simulink model "case2"  (R2024b)
settings: Solver=FixedStepAuto  StartTime=0  StopTime=1  FixedStep=1e-7  RelTol=1e-3
values from neighbouring files (symbols this model uses):
  SG_D_1_D = 0.01056    [IEEE9_case_parameters.m]    (also in case1_parameters.m; case2_parameters.m; case3_parameters.m; case4_parameters.m)
  SG_D_1_EnableSaturation = 0    [IEEE9_case_parameters.m]    (also in case1_parameters.m; case2_parameters.m; case3_parameters.m; case4_parameters.m)
  SG_D_1_f0 = 60    [IEEE9_case_parameters.m]    (also in case1_parameters.m; case2_parameters.m; case3_parameters.m; case4_parameters.m)
  SG_D_1_H = 7.5    [IEEE9_case_parameters.m]    (also in case1_parameters.m; case2_parameters.m; case3_parameters.m; case4_parameters.m)
  SG_D_1_K_A = 20    [IEEE9_case_parameters.m]    (also in case1_parameters.m; case2_parameters.m; case3_parameters.m; case4_parameters.m)
  SG_D_1_K_E = 1.000000e+1    (= 10)    [IEEE9_case_parameters.m]    (also in case1_parameters.m; case2_parameters.m; case3_parameters.m; case4_parameters.m)
  SG_D_1_K_F = 2.363    [IEEE9_case_parameters.m]    (also in case1_parameters.m; case2_parameters.m; case3_parameters.m; case4_parameters.m)
  SG_D_1_K_s = 0.5    [IEEE9_case_parameters.m]    (also in case1_parameters.m = 5; case2_parameters.m = 5; case3_parameters.m = 5; case4_parameters.m = 5)
  SG_D_1_R_a = 0.001088    [IEEE9_case_parameters.m]    (also in case1_parameters.m; case2_parameters.m; case3_parameters.m; case4_parameters.m)
  SG_D_1_S_A = 1    [IEEE9_case_parameters.m]    (also in case1_parameters.m; case2_parameters.m; case3_parameters.m; case4_parameters.m)
  SG_D_1_S_B = 0.103    [IEEE9_case_parameters.m]    (also in case1_parameters.m; case2_parameters.m; case3_parameters.m; case4_parameters.m)
  SG_D_1_S_N = 10.659857    [IEEE9_case_parameters.m]    (also in case1_parameters.m; case2_parameters.m; case3_parameters.m; case4_parameters.m)
  SG_D_1_SpeedPara = 200    [IEEE9_case_parameters.m]    (also in case1_parameters.m; case2_parameters.m; case3_parameters.m; case4_parameters.m)
  SG_D_1_T_0 = 0.720173    [IEEE9_case_parameters.m]    (also in case1_parameters.m = 0.755522; case2_parameters.m = 0.808931; case3_parameters.m = 0.869402; case4_parameters.m = 0.729316)
  SG_D_1_T_1 = 0.3    [IEEE9_case_parameters.m]    (also in case1_parameters.m; case2_parameters.m; case3_parameters.m; case4_parameters.m)
  SG_D_1_T_2 = 0.05    [IEEE9_case_parameters.m]    (also in case1_parameters.m; case2_parameters.m; case3_parameters.m; case4_parameters.m)
  SG_D_1_T_3 = 0.02    [IEEE9_case_parameters.m]    (also in case1_parameters.m; case2_parameters.m; case3_parameters.m; case4_parameters.m)
  SG_D_1_T_4 = 0.005    [IEEE9_case_parameters.m]    (also in case1_parameters.m; case2_parameters.m; case3_parameters.m; case4_parameters.m)
  SG_D_1_T_A = 0.02    [IEEE9_case_parameters.m]    (also in case1_parameters.m; case2_parameters.m; case3_parameters.m; case4_parameters.m)
  SG_D_1_T_dd = 8.000000e+0    (= 8)    [IEEE9_case_parameters.m]    (also in case1_parameters.m; case2_parameters.m; case3_parameters.m; case4_parameters.m)
  SG_D_1_T_ddd = 0.04    [IEEE9_case_parameters.m]    (also in case1_parameters.m; case2_parameters.m; case3_parameters.m; case4_parameters.m)
  SG_D_1_T_E = 0.314    [IEEE9_case_parameters.m]    (also in case1_parameters.m; case2_parameters.m; case3_parameters.m; case4_parameters.m)
  SG_D_1_T_F = 0.35    [IEEE9_case_parameters.m]    (also in case1_parameters.m; case2_parameters.m; case3_parameters.m; case4_parameters.m)
  SG_D_1_T_qd = 0.8    [IEEE9_case_parameters.m]    (also in case1_parameters.m; case2_parameters.m; case3_parameters.m; case4_parameters.m)
  SG_D_1_T_qdd = 0.02    [IEEE9_case_parameters.m]    (also in case1_parameters.m; case2_parameters.m; case3_parameters.m; case4_parameters.m)
  SG_D_1_T_speed = 0.1    [IEEE9_case_parameters.m]    (also in case1_parameters.m = 200; case2_parameters.m = 200; case3_parameters.m = 200; case4_parameters.m = 200)
  SG_D_1_T_w = 0.5    [IEEE9_case_parameters.m]    (also in case1_parameters.m; case2_parameters.m; case3_parameters.m; case4_parameters.m)
  SG_D_1_V_ref = 1.990276    [IEEE9_case_parameters.m]    (also in case1_parameters.m = 2.042296; case2_parameters.m = 2.051388; case3_parameters.m = 2.089584; case4_parameters.m = 2.01845)
  SG_D_1_w_ref = 376.991118    [IEEE9_case_parameters.m]    (also in case1_parameters.m; case2_parameters.m; case3_parameters.m; case4_parameters.m)
  SG_D_1_wb = 6.000000e+1    (= 60)    [IEEE9_case_parameters.m]    (also in case1_parameters.m; case2_parameters.m; case3_parameters.m; case4_parameters.m)
  SG_D_1_x_d = 1.9    [IEEE9_case_parameters.m]    (also in case1_parameters.m; case2_parameters.m; case3_parameters.m; case4_parameters.m)
  SG_D_1_x_dd = 0.302    [IEEE9_case_parameters.m]    (also in case1_parameters.m; case2_parameters.m; case3_parameters.m; case4_parameters.m)
  SG_D_1_x_ddd = 0.204    [IEEE9_case_parameters.m]    (also in case1_parameters.m; case2_parameters.m; case3_parameters.m; case4_parameters.m)
  SG_D_1_x_l = 0.05    [IEEE9_case_parameters.m]    (also in case1_parameters.m; case2_parameters.m; case3_parameters.m; case4_parameters.m)
  SG_D_1_x_q = 1.3    [IEEE9_case_parameters.m]    (also in case1_parameters.m; case2_parameters.m; case3_parameters.m; case4_parameters.m)
  SG_D_1_x_qd = 0.5    [IEEE9_case_parameters.m]    (also in case1_parameters.m; case2_parameters.m; case3_parameters.m; case4_parameters.m)
  SG_D_1_x_qdd = 0.3    [IEEE9_case_parameters.m]    (also in case1_parameters.m; case2_parameters.m; case3_parameters.m; case4_parameters.m)
  SG_D_2_D = 0.02    [IEEE9_case_parameters.m]    (also in case1_parameters.m; case2_parameters.m; case3_parameters.m; case4_parameters.m)
  SG_D_2_EnableSaturation = 0    [IEEE9_case_parameters.m]    (also in case1_parameters.m; case2_parameters.m; case3_parameters.m; case4_parameters.m)
  SG_D_2_f0 = 60    [IEEE9_case_parameters.m]    (also in case1_parameters.m; case2_parameters.m; case3_parameters.m; case4_parameters.m)
  SG_D_2_H = 8.000000e+0    (= 8)    [IEEE9_case_parameters.m]    (also in case1_parameters.m; case2_parameters.m; case3_parameters.m; case4_parameters.m)
  SG_D_2_K_A = 20    [IEEE9_case_parameters.m]    (also in case1_parameters.m; case2_parameters.m; case3_parameters.m; case4_parameters.m)
  SG_D_2_K_E = 1.000000e+1    (= 10)    [IEEE9_case_parameters.m]    (also in case1_parameters.m; case2_parameters.m; case3_parameters.m; case4_parameters.m)
  SG_D_2_K_F = 2.363    [IEEE9_case_parameters.m]    (also in case1_parameters.m; case2_parameters.m; case3_parameters.m; case4_parameters.m)
  SG_D_2_K_s = 0.5    [IEEE9_case_parameters.m]    (also in case1_parameters.m = 4; case2_parameters.m = 4; case3_parameters.m = 4; case4_parameters.m = 4)
  SG_D_2_R_a = 0.001088    [IEEE9_case_parameters.m]    (also in case1_parameters.m; case2_parameters.m; case3_parameters.m; case4_parameters.m)
  SG_D_2_S_A = 1    [IEEE9_case_parameters.m]    (also in case1_parameters.m; case2_parameters.m; case3_parameters.m; case4_parameters.m)
  SG_D_2_S_B = 0.103    [IEEE9_case_parameters.m]    (also in case1_parameters.m; case2_parameters.m; case3_parameters.m; case4_parameters.m)
  SG_D_2_S_N = 10.659857    [IEEE9_case_parameters.m]    (also in case1_parameters.m; case2_parameters.m; case3_parameters.m; case4_parameters.m)
  SG_D_2_SpeedPara = 200    [IEEE9_case_parameters.m]    (also in case1_parameters.m; case2_parameters.m; case3_parameters.m; case4_parameters.m)
  SG_D_2_T_0 = 1.632913    [IEEE9_case_parameters.m]    (also in case1_parameters.m = 1.632925; case2_parameters.m = 1.632915; case3_parameters.m = 1.632914; case4_parameters.m = 1.632927)
  SG_D_2_T_1 = 0.2    [IEEE9_case_parameters.m]    (also in case1_parameters.m; case2_parameters.m; case3_parameters.m; case4_parameters.m)
  SG_D_2_T_2 = 0.05    [IEEE9_case_parameters.m]    (also in case1_parameters.m; case2_parameters.m; case3_parameters.m; case4_parameters.m)
  SG_D_2_T_3 = 0.02    [IEEE9_case_parameters.m]    (also in case1_parameters.m; case2_parameters.m; case3_parameters.m; case4_parameters.m)
  SG_D_2_T_4 = 0.005    [IEEE9_case_parameters.m]    (also in case1_parameters.m; case2_parameters.m; case3_parameters.m; case4_parameters.m)
  SG_D_2_T_A = 0.02    [IEEE9_case_parameters.m]    (also in case1_parameters.m; case2_parameters.m; case3_parameters.m; case4_parameters.m)
  SG_D_2_T_dd = 7.9    [IEEE9_case_parameters.m]    (also in case1_parameters.m; case2_parameters.m; case3_parameters.m; case4_parameters.m)
  SG_D_2_T_ddd = 0.04    [IEEE9_case_parameters.m]    (also in case1_parameters.m; case2_parameters.m; case3_parameters.m; case4_parameters.m)
  SG_D_2_T_E = 0.314    [IEEE9_case_parameters.m]    (also in case1_parameters.m; case2_parameters.m; case3_parameters.m; case4_parameters.m)
  SG_D_2_T_F = 0.35    [IEEE9_case_parameters.m]    (also in case1_parameters.m; case2_parameters.m; case3_parameters.m; case4_parameters.m)
  SG_D_2_T_qd = 0.8    [IEEE9_case_parameters.m]    (also in case1_parameters.m; case2_parameters.m; case3_parameters.m; case4_parameters.m)
  SG_D_2_T_qdd = 0.015    [IEEE9_case_parameters.m]    (also in case1_parameters.m; case2_parameters.m; case3_parameters.m; case4_parameters.m)
  SG_D_2_T_speed = 0.1    [IEEE9_case_parameters.m]    (also in case1_parameters.m = 150; case2_parameters.m = 150; case3_parameters.m = 150; case4_parameters.m = 150)
  SG_D_2_T_w = 0.35    [IEEE9_case_parameters.m]    (also in case1_parameters.m; case2_parameters.m; case3_parameters.m; case4_parameters.m)
  SG_D_2_V_ref = 2.58547    [IEEE9_case_parameters.m]    (also in case1_parameters.m = 2.597896; case2_parameters.m = 2.587136; case3_parameters.m = 2.586042; case4_parameters.m = 2.599679)
  SG_D_2_w_ref = 376.991118    [IEEE9_case_parameters.m]    (also in case1_parameters.m; case2_parameters.m; case3_parameters.m; case4_parameters.m)
  SG_D_2_wb = 6.000000e+1    (= 60)    [IEEE9_case_parameters.m]    (also in case1_parameters.m; case2_parameters.m; case3_parameters.m; case4_parameters.m)
  SG_D_2_x_d = 1.8    [IEEE9_case_parameters.m]    (also in case1_parameters.m; case2_parameters.m; case3_parameters.m; case4_parameters.m)
  SG_D_2_x_dd = 0.302    [IEEE9_case_parameters.m]    (also in case1_parameters.m; case2_parameters.m; case3_parameters.m; case4_parameters.m)
  SG_D_2_x_ddd = 0.204    [IEEE9_case_parameters.m]    (also in case1_parameters.m; case2_parameters.m; case3_parameters.m; case4_parameters.m)
  SG_D_2_x_l = 0.05    [IEEE9_case_parameters.m]    (also in case1_parameters.m; case2_parameters.m; case3_parameters.m; case4_parameters.m)
  SG_D_2_x_q = 1.25    [IEEE9_case_parameters.m]    (also in case1_parameters.m; case2_parameters.m; case3_parameters.m; case4_parameters.m)
  SG_D_2_x_qd = 0.5    [IEEE9_case_parameters.m]    (also in case1_parameters.m; case2_parameters.m; case3_parameters.m; case4_parameters.m)
  SG_D_2_x_qdd = 0.3    [IEEE9_case_parameters.m]    (also in case1_parameters.m; case2_parameters.m; case3_parameters.m; case4_parameters.m)
  SG_D_3_D = 0.02    [IEEE9_case_parameters.m]    (also in case1_parameters.m; case2_parameters.m; case3_parameters.m; case4_parameters.m)
  SG_D_3_EnableSaturation = 0    [IEEE9_case_parameters.m]    (also in case1_parameters.m; case2_parameters.m; case3_parameters.m; case4_parameters.m)
  SG_D_3_f0 = 60    [IEEE9_case_parameters.m]    (also in case1_parameters.m; case2_parameters.m; case3_parameters.m; case4_parameters.m)
  SG_D_3_H = 7.7    [IEEE9_case_parameters.m]    (also in case1_parameters.m; case2_parameters.m; case3_parameters.m; case4_parameters.m)
  SG_D_3_K_A = 20    [IEEE9_case_parameters.m]    (also in case1_parameters.m; case2_parameters.m; case3_parameters.m; case4_parameters.m)
  SG_D_3_K_E = 1.000000e+1    (= 10)    [IEEE9_case_parameters.m]    (also in case1_parameters.m; case2_parameters.m; case3_parameters.m; case4_parameters.m)
  SG_D_3_K_F = 2.363    [IEEE9_case_parameters.m]    (also in case1_parameters.m; case2_parameters.m; case3_parameters.m; case4_parameters.m)
  SG_D_3_K_s = 0.2    [IEEE9_case_parameters.m]    (also in case1_parameters.m = 2; case2_parameters.m = 2; case3_parameters.m = 2; case4_parameters.m = 2)
  SG_D_3_R_a = 0.001088    [IEEE9_case_parameters.m]    (also in case1_parameters.m; case2_parameters.m; case3_parameters.m; case4_parameters.m)
  SG_D_3_S_A = 1    [IEEE9_case_parameters.m]    (also in case1_parameters.m; case2_parameters.m; case3_parameters.m; case4_parameters.m)
  SG_D_3_S_B = 0.103    [IEEE9_case_parameters.m]    (also in case1_parameters.m; case2_parameters.m; case3_parameters.m; case4_parameters.m)
  SG_D_3_S_N = 10.659857    [IEEE9_case_parameters.m]    (also in case1_parameters.m; case2_parameters.m; case3_parameters.m; case4_parameters.m)
  SG_D_3_SpeedPara = 200    [IEEE9_case_parameters.m]    (also in case1_parameters.m; case2_parameters.m; case3_parameters.m; case4_parameters.m)
  SG_D_3_T_0 = 0.850788    [IEEE9_case_parameters.m]    (also in case1_parameters.m = 0.850786; case2_parameters.m = 0.850787; case3_parameters.m; case4_parameters.m = 0.850786)
  SG_D_3_T_1 = 0.2    [IEEE9_case_parameters.m]    (also in case1_parameters.m; case2_parameters.m; case3_parameters.m; case4_parameters.m)
  SG_D_3_T_2 = 0.05    [IEEE9_case_parameters.m]    (also in case1_parameters.m; case2_parameters.m; case3_parameters.m; case4_parameters.m)
  SG_D_3_T_3 = 0.02    [IEEE9_case_parameters.m]    (also in case1_parameters.m; case2_parameters.m; case3_parameters.m; case4_parameters.m)
  SG_D_3_T_4 = 0.005    [IEEE9_case_parameters.m]    (also in case1_parameters.m; case2_parameters.m; case3_parameters.m; case4_parameters.m)
  SG_D_3_T_A = 0.02    [IEEE9_case_parameters.m]    (also in case1_parameters.m; case2_parameters.m; case3_parameters.m; case4_parameters.m)
  SG_D_3_T_dd = 8.1    [IEEE9_case_parameters.m]    (also in case1_parameters.m; case2_parameters.m; case3_parameters.m; case4_parameters.m)
  SG_D_3_T_ddd = 0.04    [IEEE9_case_parameters.m]    (also in case1_parameters.m; case2_parameters.m; case3_parameters.m; case4_parameters.m)
  SG_D_3_T_E = 0.314    [IEEE9_case_parameters.m]    (also in case1_parameters.m; case2_parameters.m; case3_parameters.m; case4_parameters.m)
  SG_D_3_T_F = 0.35    [IEEE9_case_parameters.m]    (also in case1_parameters.m; case2_parameters.m; case3_parameters.m; case4_parameters.m)
  SG_D_3_T_qd = 0.8    [IEEE9_case_parameters.m]    (also in case1_parameters.m; case2_parameters.m; case3_parameters.m; case4_parameters.m)
  SG_D_3_T_qdd = 0.015    [IEEE9_case_parameters.m]    (also in case1_parameters.m; case2_parameters.m; case3_parameters.m; case4_parameters.m)
  SG_D_3_T_speed = 0.1    [IEEE9_case_parameters.m]    (also in case1_parameters.m = 180; case2_parameters.m = 180; case3_parameters.m = 180; case4_parameters.m = 180)
  SG_D_3_T_w = 0.4    [IEEE9_case_parameters.m]    (also in case1_parameters.m; case2_parameters.m; case3_parameters.m; case4_parameters.m)
  SG_D_3_V_ref = 1.892727    [IEEE9_case_parameters.m]    (also in case1_parameters.m = 1.906439; case2_parameters.m = 1.895535; case3_parameters.m = 1.892105; case4_parameters.m = 1.906598)
  SG_D_3_w_ref = 376.991118    [IEEE9_case_parameters.m]    (also in case1_parameters.m; case2_parameters.m; case3_parameters.m; case4_parameters.m)
  SG_D_3_wb = 6.000000e+1    (= 60)    [IEEE9_case_parameters.m]    (also in case1_parameters.m; case2_parameters.m; case3_parameters.m; case4_parameters.m)
  SG_D_3_x_d = 1.85    [IEEE9_case_parameters.m]    (also in case1_parameters.m; case2_parameters.m; case3_parameters.m; case4_parameters.m)
  SG_D_3_x_dd = 0.302    [IEEE9_case_parameters.m]    (also in case1_parameters.m; case2_parameters.m; case3_parameters.m; case4_parameters.m)
  SG_D_3_x_ddd = 0.204    [IEEE9_case_parameters.m]    (also in case1_parameters.m; case2_parameters.m; case3_parameters.m; case4_parameters.m)
  SG_D_3_x_l = 0.05    [IEEE9_case_parameters.m]    (also in case1_parameters.m; case2_parameters.m; case3_parameters.m; case4_parameters.m)
  SG_D_3_x_q = 1.2    [IEEE9_case_parameters.m]    (also in case1_parameters.m; case2_parameters.m; case3_parameters.m; case4_parameters.m)
  SG_D_3_x_qd = 0.5    [IEEE9_case_parameters.m]    (also in case1_parameters.m; case2_parameters.m; case3_parameters.m; case4_parameters.m)
  SG_D_3_x_qdd = 0.3    [IEEE9_case_parameters.m]    (also in case1_parameters.m; case2_parameters.m; case3_parameters.m; case4_parameters.m)
(part 7 of 12)

== system case2/SG_D_2/T_e_SG_D_2_block ==
  note: T_e_SG_D_2 in case2
      | $-\frac{\psi _{d,\mathrm{SG},D,2}\,\left(\psi _{q,\mathrm{SG},D,2}+\frac{\psi _{\mathrm{gq},\mathrm{SG},D,2}\,\left(x_{l}-x_{\mathrm{qdd}}\right)}{x_{l}-x_{\mathrm{qd}}}+\frac{\psi _{\mathrm{kq},\mathrm{SG},D,2}\,\left(x_{\mathrm{qd}}-x_{\mathrm{qdd}}\right)}{x_{l}-x_{\mathrm{qd}}}\right)}{x_{\mathrm{qdd}}}-\frac{\psi _{q,\mathrm{SG},D,2}\,\left(\frac{\psi _{\mathrm{1d},\mathrm{SG},D,2}\,\left(x_{\mathrm{dd}}-x_{\mathrm{ddd}}\right)}{x_{\mathrm{dd}}-x_{l}}-\psi _{d,\mathrm{SG},D,2}+\frac{\psi _{\mathrm{fd},\mathrm{SG},D,2}\,\left(x_{\mathrm{ddd}}-x_{l}\right)}{x_{\mathrm{dd}}-x_{l}}\right)}{x_{\mathrm{ddd}}}$
      | Automatically generated on 2025-10-31 18:55:11 .
  State_psi_d_SG_D_2_1b998 : Inport
  State_psi_gq_SG_D_2_708b9 : Inport  Port=2
  State_psi_kq_SG_D_2_15175 : Inport  Port=3
  State_psi_q_SG_D_2_d45b5 : Inport  Port=4
  State_psi_q_SG_D_2_80989 : Inport  Port=5
  State_psi_1d_SG_D_2_98cfc : Inport  Port=6
  State_psi_d_SG_D_2_92f27 : Inport  Port=7
  State_psi_fd_SG_D_2_cd007 : Inport  Port=8
  Add_21448 : Sum
  Add_2725a : Sum
  Add_9cc90 : Sum
  Add_cd0c8 : Sum
  Add_e53d7 : Sum
  Add_ed929 : Sum
  Constant_-1_45d18 : Constant  Value=-1
  Constant_-1_6fdaf : Constant  Value=-1
  Constant_-1_b0721 : Constant  Value=-1
  Constant_-1_e149d : Constant  Value=-1
  Constant_-1_e72e6 : Constant  Value=-1
  Constant_x_dd_306b0 : Constant  Value=x_dd
  Constant_x_dd_465f3 : Constant  Value=x_dd
  Constant_x_dd_7001e : Constant  Value=x_dd
  Constant_x_ddd_5405b : Constant  Value=x_ddd
  Constant_x_ddd_794b0 : Constant  Value=x_ddd
  Constant_x_ddd_a1b47 : Constant  Value=x_ddd
  Constant_x_l_35281 : Constant  Value=x_l
  Constant_x_l_7c535 : Constant  Value=x_l
  Constant_x_l_801f4 : Constant  Value=x_l
  Constant_x_l_96b75 : Constant  Value=x_l
  Constant_x_l_a5052 : Constant  Value=x_l
  Constant_x_l_e8f25 : Constant  Value=x_l
  Constant_x_qd_228f3 : Constant  Value=x_qd
  Constant_x_qd_300e6 : Constant  Value=x_qd
  Constant_x_qd_c14fb : Constant  Value=x_qd
  Constant_x_qdd_624a4 : Constant  Value=x_qdd
  Constant_x_qdd_8f119 : Constant  Value=x_qdd
  Constant_x_qdd_bf4b0 : Constant  Value=x_qdd
  Divide_1e900 : Product  Inputs=*/
  Divide_21a18 : Product  Inputs=*/
  Divide_56f04 : Product  Inputs=*/
  Divide_8f012 : Product  Inputs=*/
  Divide_ecb2d : Product  Inputs=*/
  Divide_ffd1d : Product  Inputs=*/
  Product_021e8 : Product
  Product_2a24e : Product
  Product_3f3e5 : Product
  Product_57cca : Product
  Product_96bc8 : Product
  Product_b4c5b : Product
  Product_ba9c3 : Product
  Product_ca1fb : Product
  Product_ddd8f : Product
  Product_ebb62 : Product
  Product_fc145 : Product
  Subtract_0bcf5 : Sum  Inputs=+-
  Subtract_14a24 : Sum  Inputs=+-
  Subtract_44d98 : Sum  Inputs=+-
  Subtract_533a4 : Sum  Inputs=+-
  Subtract_5beec : Sum  Inputs=+-
  Subtract_6ff52 : Sum  Inputs=+-
  Subtract_890bb : Sum  Inputs=+-
  Blockout_T_e_SG_D_2_b8deb : Outport
  wires:
  Constant_-1_6fdaf/1 -> Product_b4c5b/1
  Divide_8f012/1 -> Subtract_44d98/1
  Constant_-1_b0721/1 -> Product_021e8/1
  Constant_x_l_801f4/1 -> Product_021e8/2
  Constant_x_qd_300e6/1 -> Subtract_890bb/1
  Product_ebb62/1 -> Divide_8f012/1
  Product_021e8/1 -> Add_21448/1
  Divide_56f04/1 -> Subtract_14a24/2
  Constant_x_qdd_bf4b0/1 -> Subtract_890bb/2
  Constant_x_qdd_8f119/1 -> Divide_1e900/2
  Constant_x_ddd_a1b47/1 -> Subtract_6ff52/2
  Constant_x_qdd_624a4/1 -> Add_21448/2
  Constant_x_l_35281/1 -> Product_b4c5b/2
  Constant_-1_e149d/1 -> Product_fc145/1
  Constant_x_l_96b75/1 -> Product_fc145/2
  Constant_-1_e72e6/1 -> Product_57cca/1
  State_psi_1d_SG_D_2_98cfc/1 -> Product_57cca/2
  Constant_x_dd_465f3/1 -> Subtract_6ff52/1
  Divide_ecb2d/1 -> Subtract_44d98/2
  State_psi_gq_SG_D_2_708b9/1 -> Product_ebb62/1
  Add_21448/1 -> Product_ebb62/2
  Subtract_44d98/1 -> Add_cd0c8/1
  Constant_x_dd_7001e/1 -> Subtract_5beec/1
  Product_b4c5b/1 -> Add_9cc90/1
  Product_3f3e5/1 -> Product_ddd8f/1
  Constant_x_qd_c14fb/1 -> Add_9cc90/2
  State_psi_kq_SG_D_2_15175/1 -> Product_ba9c3/1
  Subtract_890bb/1 -> Product_ba9c3/2
  Product_fc145/1 -> Add_ed929/1
  State_psi_q_SG_D_2_80989/1 -> Product_2a24e/1
  Constant_x_qd_228f3/1 -> Add_ed929/2
  Product_57cca/1 -> Product_96bc8/1
  Divide_21a18/1 -> Add_2725a/2
  Subtract_6ff52/1 -> Product_96bc8/2
  Constant_x_l_7c535/1 -> Subtract_5beec/2
  Constant_x_ddd_5405b/1 -> Subtract_533a4/1
  Constant_x_dd_306b0/1 -> Subtract_0bcf5/1
  Constant_x_l_a5052/1 -> Subtract_533a4/2
  Add_2725a/1 -> Blockout_T_e_SG_D_2_b8deb/1
  Add_9cc90/1 -> Divide_8f012/2
  Product_ba9c3/1 -> Divide_ecb2d/1
  Product_ddd8f/1 -> Divide_1e900/1
  State_psi_d_SG_D_2_1b998/1 -> Product_3f3e5/2
  Add_ed929/1 -> Divide_ecb2d/2
  Product_96bc8/1 -> Divide_ffd1d/1
  Subtract_5beec/1 -> Divide_ffd1d/2
  Constant_x_l_e8f25/1 -> Subtract_0bcf5/2
  State_psi_fd_SG_D_2_cd007/1 -> Product_ca1fb/1
  Constant_x_ddd_794b0/1 -> Divide_21a18/2
  Product_2a24e/1 -> Divide_21a18/1
  Subtract_533a4/1 -> Product_ca1fb/2
  Divide_ffd1d/1 -> Add_e53d7/1
  State_psi_d_SG_D_2_92f27/1 -> Add_e53d7/2
  Add_e53d7/1 -> Subtract_14a24/1
  Product_ca1fb/1 -> Divide_56f04/1
  Subtract_0bcf5/1 -> Divide_56f04/2
  Constant_-1_45d18/1 -> Product_3f3e5/1
  State_psi_q_SG_D_2_d45b5/1 -> Add_cd0c8/2
  Add_cd0c8/1 -> Product_ddd8f/2
  Subtract_14a24/1 -> Product_2a24e/2
  Divide_1e900/1 -> Add_2725a/1

== system case2/SG_D_2/d_E_fd_SG_D_2_block ==
  note: d_E_fd_SG_D_2 in case2
      | $\frac{V_{f,\mathrm{SG},D,2}-E_{\mathrm{fd},\mathrm{SG},D,2}\,K_{E}}{T_{E}}$
      | Automatically generated on 2025-10-31 18:54:53 .
  State_E_fd_SG_D_2_04f17 : Inport
  State_V_f_SG_D_2_edff6 : Inport  Port=2
  Add_1eb67 : Sum
  Constant_-1_fcf40 : Constant  Value=-1
  Constant_K_E_77049 : Constant  Value=K_E
  Constant_T_E_b4b89 : Constant  Value=T_E
  Divide_daa25 : Product  Inputs=*/
  Product_c6f6a : Product
  Product_d4e76 : Product
  Blockout_d_E_fd_SG_D_2_d404e : Outport
  wires:
  Constant_-1_fcf40/1 -> Product_d4e76/1
  State_E_fd_SG_D_2_04f17/1 -> Product_d4e76/2
  Product_d4e76/1 -> Product_c6f6a/1
  Constant_K_E_77049/1 -> Product_c6f6a/2
  Product_c6f6a/1 -> Add_1eb67/1
  Constant_T_E_b4b89/1 -> Divide_daa25/2
  State_V_f_SG_D_2_edff6/1 -> Add_1eb67/2
  Add_1eb67/1 -> Divide_daa25/1
  Divide_daa25/1 -> Blockout_d_E_fd_SG_D_2_d404e/1

== system case2/SG_D_2/d_Px_1_SG_D_2_block ==
  note: d_Px_1_SG_D_2 in case2
      | $\frac{w_{\mathrm{SG},D,2}-2\,\pi \,f_{0}}{T_{w}}-\frac{\mathrm{Px}_{1,\mathrm{SG},D,2}}{T_{w}}$
      | Automatically generated on 2025-10-31 18:54:54 .
  State_Px_1_SG_D_2_d590c : Inport
  State_w_SG_D_2_84017 : Inport  Port=2
  Add_2d97d : Sum
  Add_5b859 : Sum
  Constant_-1_e7105 : Constant  Value=-1
  Constant_-2.0_87bde : Constant  Value=-2.0
  Constant_T_w_0e214 : Constant  Value=T_w
  Constant_T_w_b2a2b : Constant  Value=T_w
  Constant_f0_fd3df : Constant  Value=f0
  Constant_pi_fb42a : Constant  Value=pi
  Divide_6014e : Product  Inputs=*/
  Divide_b64ea : Product  Inputs=*/
  Product_56379 : Product
  Product_68060 : Product
  Product_fcbc4 : Product
  Blockout_d_Px_1_SG_D_2_b8a6d : Outport
  wires:
  Constant_-2.0_87bde/1 -> Product_56379/1
  State_w_SG_D_2_84017/1 -> Add_5b859/2
  Constant_pi_fb42a/1 -> Product_56379/2
  Product_56379/1 -> Product_fcbc4/1
  Constant_f0_fd3df/1 -> Product_fcbc4/2
  Constant_-1_e7105/1 -> Product_68060/1
  State_Px_1_SG_D_2_d590c/1 -> Product_68060/2
  Product_fcbc4/1 -> Add_5b859/1
  Product_68060/1 -> Divide_6014e/1
  Constant_T_w_0e214/1 -> Divide_6014e/2
  Add_5b859/1 -> Divide_b64ea/1
  Constant_T_w_b2a2b/1 -> Divide_b64ea/2
  Divide_6014e/1 -> Add_2d97d/1
  Divide_b64ea/1 -> Add_2d97d/2
  Add_2d97d/1 -> Blockout_d_Px_1_SG_D_2_b8a6d/1

== system case2/SG_D_2/d_Px_2_SG_D_2_block ==
  note: d_Px_2_SG_D_2 in case2
      | $\frac{\mathrm{Px}_{1,\mathrm{SG},D,2}-T_{2}\,\left(\frac{\mathrm{Px}_{1,\mathrm{SG},D,2}}{T_{w}}-\frac{w_{\mathrm{SG},D,2}-2\,\pi \,f_{0}}{T_{w}}\right)}{T_{1}}-\frac{\mathrm{Px}_{2,\mathrm{SG},D,2}}{T_{1}}$
      | Automatically generated on 2025-10-31 18:54:56 .
  State_Px_2_SG_D_2_f980a : Inport
  State_Px_1_SG_D_2_3257e : Inport  Port=2
  State_Px_1_SG_D_2_9c84f : Inport  Port=3
  State_w_SG_D_2_45781 : Inport  Port=4
  Add_239d6 : Sum
  Add_9d82b : Sum
  Add_a15b9 : Sum
  Add_afd59 : Sum
  Constant_-1_7777e : Constant  Value=-1
  Constant_-1_cf267 : Constant  Value=-1
  Constant_-2.0_189ce : Constant  Value=-2.0
  Constant_T_1_a4d40 : Constant  Value=T_1
  Constant_T_1_ec3c8 : Constant  Value=T_1
  Constant_T_2_292f6 : Constant  Value=T_2
  Constant_T_w_379af : Constant  Value=T_w
  Constant_T_w_b7016 : Constant  Value=T_w
  Constant_f0_2357a : Constant  Value=f0
  Constant_pi_7038f : Constant  Value=pi
  Divide_524e1 : Product  Inputs=*/
  Divide_58d27 : Product  Inputs=*/
  Divide_8e8cc : Product  Inputs=*/
  Divide_d9104 : Product  Inputs=*/
  Product_0a6a0 : Product
  Product_325fb : Product
  Product_92f91 : Product
  Product_bc358 : Product
  Product_e1935 : Product
  Blockout_d_Px_2_SG_D_2_22689 : Outport
  wires:
  Constant_-1_7777e/1 -> Product_92f91/1
  Constant_-2.0_189ce/1 -> Product_bc358/1
  Product_0a6a0/1 -> Add_a15b9/2
  State_w_SG_D_2_45781/1 -> Add_9d82b/2
  Constant_pi_7038f/1 -> Product_bc358/2
  Product_bc358/1 -> Product_e1935/1
  State_Px_1_SG_D_2_9c84f/1 -> Product_325fb/2
  Constant_f0_2357a/1 -> Product_e1935/2
  State_Px_2_SG_D_2_f980a/1 -> Product_92f91/2
  Constant_-1_cf267/1 -> Product_325fb/1
  Product_e1935/1 -> Add_9d82b/1
  Product_325fb/1 -> Divide_8e8cc/1
  Constant_T_w_b7016/1 -> Divide_8e8cc/2
  Add_9d82b/1 -> Divide_58d27/1
  Constant_T_w_379af/1 -> Divide_58d27/2
  Divide_8e8cc/1 -> Add_239d6/1
  Divide_58d27/1 -> Add_239d6/2
  Constant_T_2_292f6/1 -> Product_0a6a0/1
  Add_239d6/1 -> Product_0a6a0/2
  State_Px_1_SG_D_2_3257e/1 -> Add_a15b9/1
  Product_92f91/1 -> Divide_d9104/1
  Constant_T_1_a4d40/1 -> Divide_d9104/2
  Add_a15b9/1 -> Divide_524e1/1
  Constant_T_1_ec3c8/1 -> Divide_524e1/2
  Divide_d9104/1 -> Add_afd59/1
  Divide_524e1/1 -> Add_afd59/2
  Add_afd59/1 -> Blockout_d_Px_2_SG_D_2_22689/1

== system case2/SG_D_2/d_Px_3_SG_D_2_block ==
  note: d_Px_3_SG_D_2 in case2
      | $\frac{\mathrm{Px}_{2,\mathrm{SG},D,2}+T_{4}\,\left(\frac{\mathrm{Px}_{1,\mathrm{SG},D,2}-T_{2}\,\left(\frac{\mathrm{Px}_{1,\mathrm{SG},D,2}}{T_{w}}-\frac{w_{\mathrm{SG},D,2}-2\,\pi \,f_{0}}{T_{w}}\right)}{T_{1}}-\frac{\mathrm{Px}_{2,\mathrm{SG},D,2}}{T_{1}}\right)}{T_{3}}-\frac{\mathrm{Px}_{3,\mathrm{SG},D,2}}{T_{3}}$
      | Automatically generated on 2025-10-31 18:54:59 .
  State_Px_3_SG_D_2_650ae : Inport
  State_Px_2_SG_D_2_61639 : Inport  Port=2
  State_Px_2_SG_D_2_4e1b7 : Inport  Port=3
  State_Px_1_SG_D_2_cef04 : Inport  Port=4
  State_Px_1_SG_D_2_2a306 : Inport  Port=5
  State_w_SG_D_2_38541 : Inport  Port=6
  Add_0ee48 : Sum
  Add_57b18 : Sum
  Add_6c6d7 : Sum
  Add_760ca : Sum
  Add_7d821 : Sum
  Add_d5425 : Sum
  Constant_-1_2e553 : Constant  Value=-1
  Constant_-1_2f7cd : Constant  Value=-1
  Constant_-1_328bc : Constant  Value=-1
  Constant_-2.0_9399b : Constant  Value=-2.0
  Constant_T_1_0d622 : Constant  Value=T_1
  Constant_T_1_add60 : Constant  Value=T_1
  Constant_T_2_a937c : Constant  Value=T_2
  Constant_T_3_37e44 : Constant  Value=T_3
  Constant_T_3_ded95 : Constant  Value=T_3
  Constant_T_4_99d81 : Constant  Value=T_4
  Constant_T_w_a9bca : Constant  Value=T_w
  Constant_T_w_c8446 : Constant  Value=T_w
  Constant_f0_f2bf7 : Constant  Value=f0
  Constant_pi_ff522 : Constant  Value=pi
  Divide_041cc : Product  Inputs=*/
  Divide_4a8b9 : Product  Inputs=*/
  Divide_5d59b : Product  Inputs=*/
  Divide_5f4cc : Product  Inputs=*/
  Divide_767e3 : Product  Inputs=*/
  Divide_8159a : Product  Inputs=*/
  Product_03317 : Product
  Product_09cb1 : Product
  Product_3ff70 : Product
  Product_6633c : Product
  Product_8eef1 : Product
  Product_9c7e0 : Product
  Product_ad926 : Product
  Blockout_d_Px_3_SG_D_2_0a542 : Outport
  wires:
  Constant_-2.0_9399b/1 -> Product_03317/1
  State_w_SG_D_2_38541/1 -> Add_0ee48/2
  Add_57b18/1 -> Divide_5f4cc/1
  Constant_pi_ff522/1 -> Product_03317/2
  Constant_-1_2e553/1 -> Product_8eef1/1
  Product_03317/1 -> Product_3ff70/1
  State_Px_2_SG_D_2_4e1b7/1 -> Product_8eef1/2
  State_Px_1_SG_D_2_2a306/1 -> Product_09cb1/2
  Divide_5f4cc/1 -> Add_760ca/2
  Constant_f0_f2bf7/1 -> Product_3ff70/2
  Constant_-1_328bc/1 -> Product_09cb1/1
  Product_3ff70/1 -> Add_0ee48/1
  Product_09cb1/1 -> Divide_041cc/1
  Constant_T_w_c8446/1 -> Divide_041cc/2
  Divide_8159a/1 -> Add_760ca/1
  Add_0ee48/1 -> Divide_767e3/1
  Product_9c7e0/1 -> Add_d5425/2
  Constant_T_w_a9bca/1 -> Divide_767e3/2
  Divide_041cc/1 -> Add_7d821/1
  State_Px_1_SG_D_2_cef04/1 -> Add_d5425/1
  Divide_767e3/1 -> Add_7d821/2
  Constant_-1_2f7cd/1 -> Product_6633c/1
  Constant_T_2_a937c/1 -> Product_9c7e0/1
  Add_7d821/1 -> Product_9c7e0/2
  Product_8eef1/1 -> Divide_5d59b/1
  Constant_T_1_0d622/1 -> Divide_5d59b/2
  Add_d5425/1 -> Divide_4a8b9/1
  Constant_T_1_add60/1 -> Divide_4a8b9/2
  Divide_5d59b/1 -> Add_6c6d7/1
  Divide_4a8b9/1 -> Add_6c6d7/2
  Constant_T_4_99d81/1 -> Product_ad926/1
  Add_6c6d7/1 -> Product_ad926/2
  State_Px_3_SG_D_2_650ae/1 -> Product_6633c/2
  State_Px_2_SG_D_2_61639/1 -> Add_57b18/1
  Product_ad926/1 -> Add_57b18/2
  Product_6633c/1 -> Divide_8159a/1
  Constant_T_3_37e44/1 -> Divide_8159a/2
  Constant_T_3_ded95/1 -> Divide_5f4cc/2
  Add_760ca/1 -> Blockout_d_Px_3_SG_D_2_0a542/1

== system case2/SG_D_2/d_R_f_SG_D_2_block ==
  note: d_R_f_SG_D_2 in case2
      | $-\frac{R_{f,\mathrm{SG},D,2}-\frac{E_{\mathrm{fd},\mathrm{SG},D,2}\,K_{F}}{T_{F}}}{T_{F}}$
      | Automatically generated on 2025-10-31 18:54:52 .
  State_E_fd_SG_D_2_001ad : Inport
  State_R_f_SG_D_2_5b4f1 : Inport  Port=2
  Constant_K_F_6271d : Constant  Value=K_F
  Constant_T_F_5f6f2 : Constant  Value=T_F
  Constant_T_F_a126e : Constant  Value=T_F
  Divide_332c4 : Product  Inputs=*/
  Divide_94a5c : Product  Inputs=*/
  Product_30b13 : Product
  Subtract_37223 : Sum  Inputs=+-
  Blockout_d_R_f_SG_D_2_fdb54 : Outport
  wires:
  Constant_T_F_a126e/1 -> Divide_332c4/2
  State_E_fd_SG_D_2_001ad/1 -> Product_30b13/1
  Constant_K_F_6271d/1 -> Product_30b13/2
  State_R_f_SG_D_2_5b4f1/1 -> Subtract_37223/2
  Product_30b13/1 -> Divide_332c4/1
  Divide_332c4/1 -> Subtract_37223/1
  Constant_T_F_5f6f2/1 -> Divide_94a5c/2
  Subtract_37223/1 -> Divide_94a5c/1
  Divide_94a5c/1 -> Blockout_d_R_f_SG_D_2_fdb54/1

== system case2/SG_D_2/d_T_m_SG_D_2_block ==
  note: d_T_m_SG_D_2 in case2
      | $-\frac{T_{m,\mathrm{SG},D,2}-T_{0}+\frac{\mathrm{SpeedPara}\,\left(w_{\mathrm{SG},D,2}-w_{\mathrm{ref}}\right)}{2\,f_{0}\,\pi }}{T_{\mathrm{speed}}}$
      | Automatically generated on 2025-10-31 18:54:42 .
  State_w_SG_D_2_14e8c : Inport
  State_T_m_SG_D_2_165ac : Inport  Port=2
  Add_59356 : Sum
  Add_e3ccf : Sum
  Constant_-1_18455 : Constant  Value=-1
  Constant_2.0_d947b : Constant  Value=2.0
  Constant_SpeedPara_4386a : Constant  Value=SpeedPara
  Constant_T_0_96a28 : Constant  Value=T_0
  Constant_T_speed_188b9 : Constant  Value=T_speed
  Constant_f0_d099e : Constant  Value=f0
  Constant_pi_440c3 : Constant  Value=pi
  Constant_w_ref_23e06 : Constant  Value=w_ref
  Divide_c7a99 : Product  Inputs=*/
  Divide_f81af : Product  Inputs=*/
  Product_4d393 : Product
  Product_95a54 : Product
  Product_9dc07 : Product
  Product_c6d32 : Product
  Subtract_b1096 : Sum  Inputs=+-
  Blockout_d_T_m_SG_D_2_4b089 : Outport
  wires:
  Constant_pi_440c3/1 -> Product_95a54/2
  Constant_-1_18455/1 -> Product_4d393/1
  Constant_w_ref_23e06/1 -> Add_e3ccf/2
  State_w_SG_D_2_14e8c/1 -> Product_4d393/2
  Product_4d393/1 -> Add_e3ccf/1
  Add_59356/1 -> Subtract_b1096/1
  Add_e3ccf/1 -> Product_c6d32/2
  Constant_2.0_d947b/1 -> Product_95a54/1
  Constant_SpeedPara_4386a/1 -> Product_c6d32/1
  Product_95a54/1 -> Product_9dc07/1
  Constant_f0_d099e/1 -> Product_9dc07/2
  Product_c6d32/1 -> Divide_f81af/1
  Product_9dc07/1 -> Divide_f81af/2
  Divide_f81af/1 -> Add_59356/1
  Constant_T_0_96a28/1 -> Add_59356/2
  State_T_m_SG_D_2_165ac/1 -> Subtract_b1096/2
  Subtract_b1096/1 -> Divide_c7a99/1
  Constant_T_speed_188b9/1 -> Divide_c7a99/2
  Divide_c7a99/1 -> Blockout_d_T_m_SG_D_2_4b089/1

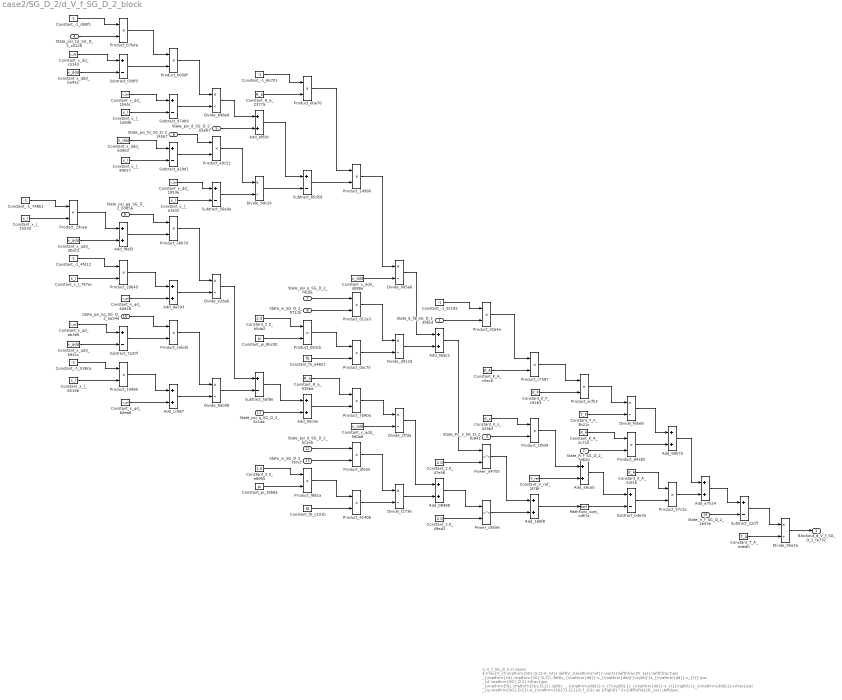
== system case2/SG_D_2/d_V_f_SG_D_2_block ==
  note: d_V_f_SG_D_2 in case2
      | $-\frac{V_{f,\mathrm{SG},D,2}-K_{A}\,\left(V_{\mathrm{ref}}-\sqrt{{\left(\frac{R_{a}\,\left(\frac{\psi _{\mathrm{1d},\mathrm{SG},D,2}\,\left(x_{\mathrm{dd}}-x_{\mathrm{ddd}}\right)}{x_{\mathrm{dd}}-x_{l}}-\psi _{d,\mathrm{SG},D,2}+\frac{\psi _{\mathrm{fd},\mathrm{SG},D,2}\,\left(x_{\mathrm{ddd}}-x_{l}\right)}{x_{\mathrm{dd}}-x_{l}}\right)}{x_{\mathrm{ddd}}}+\frac{\psi _{q,\mathrm{SG},D,2}\,w_{\mathrm{SG},D,2}}{2\,f_{0}\,\pi }\right)}^2+{\left(\frac{R_{a}\,\left(\psi _{q,\mathrm{SG},D,2}+\frac{\psi _{\mathrm{gq},\mathrm{SG},D,2}\,\left(x_{l}-x_{\mathrm{qdd}}\right)}{x_{l}-x_{\mathrm{qd}}}+\frac{\psi _{\mathrm{kq},\mathrm{SG},D,2}\,\left(x_{\mathrm{qd}}-x_{\mathrm{qdd}}\right)}{x_{l}-x_{\mathrm{qd}}}\right)}{x_{\mathrm{qdd}}}+\frac{\psi _{d,\mathrm{SG},D,2}\,w_{\mathrm{SG},D,2}}{2\,f_{0}\,\pi }\right)}^2}+K_{s}\,\mathrm{Px}_{3,\mathrm{SG},D,2}\right)-K_{A}\,R_{f,\mathrm{SG},D,2}+\frac{E_{\mathrm{fd},\mathrm{SG},D,2}\,K_{A}\,K_{F}}{T_{F}}}{T_{A}}$
      | Automatically generated on 2025-10-31 18:54:50 .
  State_E_fd_SG_D_2_39bcd : Inport
  State_R_f_SG_D_2_7d620 : Inport  Port=2
  State_Px_3_SG_D_2_fb941 : Inport  Port=3
  State_psi_1d_SG_D_2_c0128 : Inport  Port=4
  State_psi_d_SG_D_2_b5e07 : Inport  Port=5
  State_psi_fd_SG_D_2_145b7 : Inport  Port=6
  State_psi_q_SG_D_2_f4c0e : Inport  Port=7
  State_w_SG_D_2_9712b : Inport  Port=8
  State_psi_gq_SG_D_2_6385a : Inport  Port=9
  State_psi_kq_SG_D_2_aa54e : Inport  Port=10
  State_psi_q_SG_D_2_6c1aa : Inport  Port=11
  State_psi_d_SG_D_2_bc1e6 : Inport  Port=12
  State_w_SG_D_2_f97cf : Inport  Port=13
  State_V_f_SG_D_2_2e53e : Inport  Port=14
  Add_00c9e : Sum
  Add_08498 : Sum
  Add_166f8 : Sum
  Add_5b6c1 : Sum
  Add_69b7b : Sum
  Add_9a593 : Sum
  Add_a6cab : Sum
  Add_cc987 : Sum
  Add_e7524 : Sum
  Add_ef83c : Sum
  Add_f8ef2 : Sum
  Constant_-1_4fd12 : Constant  Value=-1
  Constant_-1_538ca : Constant  Value=-1
  Constant_-1_6b701 : Constant  Value=-1
  Constant_-1_6c192 : Constant  Value=-1
  Constant_-1_748b1 : Constant  Value=-1
  Constant_-1_db8f1 : Constant  Value=-1
  Constant_2.0_47e56 : Constant  Value=2.0
  Constant_2.0_49ad2 : Constant  Value=2.0
  Constant_2.0_b5da2 : Constant  Value=2.0
  Constant_2.0_e8995 : Constant  Value=2.0
  Constant_K_A_2c710 : Constant  Value=K_A
  Constant_K_A_52f16 : Constant  Value=K_A
  Constant_K_A_c5ec6 : Constant  Value=K_A
  Constant_K_F_c92b3 : Constant  Value=K_F
  Constant_K_s_029b3 : Constant  Value=K_s
  Constant_R_a_2377a : Constant  Value=R_a
  Constant_R_a_939ba : Constant  Value=R_a
  Constant_T_A_eded0 : Constant  Value=T_A
  Constant_T_F_3b21c : Constant  Value=T_F
  Constant_V_ref_2f76f : Constant  Value=V_ref
  Constant_f0_a4822 : Constant  Value=f0
  Constant_f0_c231b : Constant  Value=f0
  Constant_pi_18b8a : Constant  Value=pi
  Constant_pi_8bc00 : Constant  Value=pi
  Constant_x_dd_1953e : Constant  Value=x_dd
  Constant_x_dd_1b65c : Constant  Value=x_dd
  Constant_x_dd_c5143 : Constant  Value=x_dd
  Constant_x_ddd_63d63 : Constant  Value=x_ddd
  Constant_x_ddd_be452 : Constant  Value=x_ddd
  Constant_x_ddd_d088e : Constant  Value=x_ddd
  Constant_x_l_1a8d6 : Constant  Value=x_l
  Constant_x_l_25530 : Constant  Value=x_l
  Constant_x_l_787ec : Constant  Value=x_l
  Constant_x_l_8219b : Constant  Value=x_l
  Constant_x_l_84017 : Constant  Value=x_l
  Constant_x_l_e1632 : Constant  Value=x_l
  Constant_x_qd_40d28 : Constant  Value=x_qd
  Constant_x_qd_ab3e6 : Constant  Value=x_qd
  Constant_x_qd_b0ea6 : Constant  Value=x_qd
  Constant_x_qdd_30dc3 : Constant  Value=x_qdd
  Constant_x_qdd_560a8 : Constant  Value=x_qdd
  Constant_x_qdd_6941c : Constant  Value=x_qdd
  Divide_005e6 : Product  Inputs=*/
  Divide_2ffda : Product  Inputs=*/
  Divide_8ab08 : Product  Inputs=*/
  Divide_95e2a : Product  Inputs=*/
  Divide_9dc24 : Product  Inputs=*/
  Divide_b98e8 : Product  Inputs=*/
  Divide_d912d : Product  Inputs=*/
  Divide_e26eb : Product  Inputs=*/
  Divide_f2736 : Product  Inputs=*/
  Divide_f65e8 : Product  Inputs=*/
  MathFunc_sqrt_cd67a : Sqrt
  Power_c8a56 : Math  Operator=pow
  Power_d4705 : Math  Operator=pow
  Product_063cb : Product
  Product_0ba70 : Product
  Product_{14996,19485,41406,64282} (4 alike) : Product
  Product_1f839 : Product
  Product_29caa : Product
  Product_2bb7d : Product
  Product_2d649 : Product
  Product_32a4e : Product
  Product_57c2a : Product
  Product_7b90a : Product
  Product_a9c52 : Product
  Product_b03df : Product
  Product_b7b4a : Product
  Product_c7587 : Product
  Product_cebdd : Product
  Product_d12a3 : Product
  Product_dac75 : Product
  Product_dfe55 : Product
  Product_ecf53 : Product
  Product_f861a : Product
  Subtract_039f3 : Sum  Inputs=+-
  Subtract_22cff : Sum  Inputs=+-
  Subtract_56e0e : Sum  Inputs=+-
  Subtract_5af8e : Sum  Inputs=+-
  Subtract_7a20f : Sum  Inputs=+-
  Subtract_85d59 : Sum  Inputs=+-
  Subtract_a18d1 : Sum  Inputs=+-
  Subtract_bde3a : Sum  Inputs=+-
  Subtract_d74b9 : Sum  Inputs=+-
  Blockout_d_V_f_SG_D_2_fa732 : Outport
  wires:
  Constant_-1_db8f1/1 -> Product_b7b4a/1
  Constant_2.0_b5da2/1 -> Product_063cb/1
  Constant_-1_748b1/1 -> Product_29caa/1
  Product_063cb/1 -> Product_dac75/1
  Product_29caa/1 -> Add_f8ef2/1
  Constant_x_l_8219b/1 -> Product_19485/2
  Constant_x_l_25530/1 -> Product_29caa/2
  State_psi_1d_SG_D_2_c0128/1 -> Product_b7b4a/2
  Constant_x_l_e1632/1 -> Subtract_56e0e/2
  Constant_x_dd_c5143/1 -> Subtract_039f3/1
  Product_7b90a/1 -> Divide_2ffda/1
  Constant_x_ddd_be452/1 -> Subtract_039f3/2
  Constant_x_qd_b0ea6/1 -> Add_cc987/2
  Add_f8ef2/1 -> Product_2bb7d/2
  Constant_x_qdd_30dc3/1 -> Add_f8ef2/2
  Constant_-1_4fd12/1 -> Product_2d649/1
  Constant_x_dd_1953e/1 -> Subtract_56e0e/1
  Subtract_5af8e/1 -> Add_00c9e/1
  Power_d4705/1 -> Add_166f8/1
  Constant_x_l_787ec/1 -> Product_2d649/2
  Constant_2.0_e8995/1 -> Product_f861a/1
  Constant_x_qd_ab3e6/1 -> Subtract_7a20f/1
  Constant_pi_18b8a/1 -> Product_f861a/2
  Subtract_85d59/1 -> Product_14996/2
  Constant_x_qdd_6941c/1 -> Subtract_7a20f/2
  State_psi_fd_SG_D_2_145b7/1 -> Product_a9c52/1
  Constant_-1_538ca/1 -> Product_19485/1
  Product_b7b4a/1 -> Product_b03df/1
  State_w_SG_D_2_f97cf/1 -> Product_dfe55/2
  Subtract_039f3/1 -> Product_b03df/2
  Constant_x_dd_1b65c/1 -> Subtract_d74b9/1
  State_psi_q_SG_D_2_6c1aa/1 -> Add_00c9e/2
  State_w_SG_D_2_9712b/1 -> Product_d12a3/2
  Subtract_a18d1/1 -> Product_a9c52/2
  Constant_x_l_1a8d6/1 -> Subtract_d74b9/2
  Add_69b7b/1 -> Add_e7524/1
  Constant_x_ddd_63d63/1 -> Subtract_a18d1/1
  Constant_x_l_84017/1 -> Subtract_a18d1/2
  State_psi_gq_SG_D_2_6385a/1 -> Product_2bb7d/1
  Product_2d649/1 -> Add_9a593/1
  Subtract_56e0e/1 -> Divide_9dc24/2
  Constant_x_qd_40d28/1 -> Add_9a593/2
  Product_d12a3/1 -> Divide_d912d/1
  State_psi_kq_SG_D_2_aa54e/1 -> Product_cebdd/1
  Subtract_7a20f/1 -> Product_cebdd/2
  Product_a9c52/1 -> Divide_9dc24/1
  State_V_f_SG_D_2_2e53e/1 -> Subtract_22cff/2
  Product_19485/1 -> Add_cc987/1
  Product_b03df/1 -> Divide_b98e8/1
  Divide_e26eb/1 -> Subtract_5af8e/1
  Subtract_d74b9/1 -> Divide_b98e8/2
  Product_2bb7d/1 -> Divide_e26eb/1
  Add_9a593/1 -> Divide_e26eb/2
  Product_cebdd/1 -> Divide_8ab08/1
  Divide_9dc24/1 -> Subtract_85d59/2
  Constant_f0_a4822/1 -> Product_dac75/2
  Add_cc987/1 -> Divide_8ab08/2
  Divide_b98e8/1 -> Add_ef83c/1
  State_psi_d_SG_D_2_b5e07/1 -> Add_ef83c/2
  Divide_8ab08/1 -> Subtract_5af8e/2
  Constant_-1_6b701/1 -> Product_0ba70/1
  Constant_R_a_2377a/1 -> Product_0ba70/2
  Constant_f0_c231b/1 -> Product_41406/2
  Add_ef83c/1 -> Subtract_85d59/1
  Product_0ba70/1 -> Product_14996/1
  Constant_pi_8bc00/1 -> Product_063cb/2
  State_psi_q_SG_D_2_f4c0e/1 -> Product_d12a3/1
  Constant_R_a_939ba/1 -> Product_7b90a/1
  State_E_fd_SG_D_2_39bcd/1 -> Product_32a4e/2
  Add_00c9e/1 -> Product_7b90a/2
  State_psi_d_SG_D_2_bc1e6/1 -> Product_dfe55/1
  Product_f861a/1 -> Product_41406/1
  Product_14996/1 -> Divide_005e6/1
  Constant_x_ddd_d088e/1 -> Divide_005e6/2
  Product_dac75/1 -> Divide_d912d/2
  Constant_x_qdd_560a8/1 -> Divide_2ffda/2
  Product_dfe55/1 -> Divide_f2736/1
  Product_41406/1 -> Divide_f2736/2
  Divide_005e6/1 -> Add_5b6c1/1
  Divide_d912d/1 -> Add_5b6c1/2
  Divide_2ffda/1 -> Add_08498/1
  Divide_f2736/1 -> Add_08498/2
  Constant_-1_6c192/1 -> Product_32a4e/1
  Add_5b6c1/1 -> Power_d4705/1
  Constant_2.0_47e56/1 -> Power_d4705/2
  Add_08498/1 -> Power_c8a56/1
  Constant_2.0_49ad2/1 -> Power_c8a56/2
  Product_32a4e/1 -> Product_c7587/1
  Constant_K_A_c5ec6/1 -> Product_c7587/2
  Constant_K_s_029b3/1 -> Product_1f839/1
  State_Px_3_SG_D_2_fb941/1 -> Product_1f839/2
  Power_c8a56/1 -> Add_166f8/2
  Product_c7587/1 -> Product_ecf53/1
  Constant_K_F_c92b3/1 -> Product_ecf53/2
  Product_1f839/1 -> Add_a6cab/1
  Constant_V_ref_2f76f/1 -> Add_a6cab/2
  Add_166f8/1 -> MathFunc_sqrt_cd67a/1
  Product_ecf53/1 -> Divide_f65e8/1
  Constant_T_F_3b21c/1 -> Divide_f65e8/2
  Constant_K_A_2c710/1 -> Product_64282/1
  State_R_f_SG_D_2_7d620/1 -> Product_64282/2
  Add_a6cab/1 -> Subtract_bde3a/1
  MathFunc_sqrt_cd67a/1 -> Subtract_bde3a/2
  Divide_f65e8/1 -> Add_69b7b/1
  Product_64282/1 -> Add_69b7b/2
  Constant_K_A_52f16/1 -> Product_57c2a/1
  Subtract_bde3a/1 -> Product_57c2a/2
  Product_57c2a/1 -> Add_e7524/2
  Add_e7524/1 -> Subtract_22cff/1
  Subtract_22cff/1 -> Divide_95e2a/1
  Constant_T_A_eded0/1 -> Divide_95e2a/2
  Divide_95e2a/1 -> Blockout_d_V_f_SG_D_2_fa732/1

== system case2/SG_D_2/d_psi_1d_SG_D_2_block ==
  note: d_psi_1d_SG_D_2 in case2
      | $-\frac{\psi _{\mathrm{1d},\mathrm{SG},D,2}-\psi _{\mathrm{fd},\mathrm{SG},D,2}+\frac{\left(x_{\mathrm{dd}}-x_{l}\right)\,\left(\frac{\psi _{\mathrm{1d},\mathrm{SG},D,2}\,\left(x_{\mathrm{dd}}-x_{\mathrm{ddd}}\right)}{x_{\mathrm{dd}}-x_{l}}-\psi _{d,\mathrm{SG},D,2}+\frac{\psi _{\mathrm{fd},\mathrm{SG},D,2}\,\left(x_{\mathrm{ddd}}-x_{l}\right)}{x_{\mathrm{dd}}-x_{l}}\right)}{x_{\mathrm{ddd}}}}{T_{\mathrm{ddd}}}$
      | Automatically generated on 2025-10-31 18:54:24 .
  State_psi_1d_SG_D_2_7ee43 : Inport
  State_psi_fd_SG_D_2_21e47 : Inport  Port=2
  State_psi_1d_SG_D_2_6e6f3 : Inport  Port=3
  State_psi_d_SG_D_2_2e599 : Inport  Port=4
  State_psi_fd_SG_D_2_221ae : Inport  Port=5
  Add_0985b : Sum
  Add_8c972 : Sum
  Add_e30b2 : Sum
  Constant_-1_ac0c6 : Constant  Value=-1
  Constant_-1_b3346 : Constant  Value=-1
  Constant_T_ddd_fa46a : Constant  Value=T_ddd
  Constant_x_dd_0e8be : Constant  Value=x_dd
  Constant_x_dd_70482 : Constant  Value=x_dd
  Constant_x_dd_b4462 : Constant  Value=x_dd
  Constant_x_dd_e3a6e : Constant  Value=x_dd
  Constant_x_ddd_69af6 : Constant  Value=x_ddd
  Constant_x_ddd_7a908 : Constant  Value=x_ddd
  Constant_x_ddd_a8d87 : Constant  Value=x_ddd
  Constant_x_l_18580 : Constant  Value=x_l
  Constant_x_l_3de7a : Constant  Value=x_l
  Constant_x_l_fd65c : Constant  Value=x_l
  Constant_x_l_fe476 : Constant  Value=x_l
  Divide_4ce7a : Product  Inputs=*/
  Divide_4f7f4 : Product  Inputs=*/
  Divide_ed9f4 : Product  Inputs=*/
  Divide_f76fa : Product  Inputs=*/
  Product_20c61 : Product
  Product_4e370 : Product
  Product_802e4 : Product
  Product_97c58 : Product
  Product_cf416 : Product
  Subtract_0d414 : Sum  Inputs=+-
  Subtract_4d5aa : Sum  Inputs=+-
  Subtract_50a4c : Sum  Inputs=+-
  Subtract_a8385 : Sum  Inputs=+-
  Subtract_c1786 : Sum  Inputs=+-
  Subtract_f99a1 : Sum  Inputs=+-
  Blockout_d_psi_1d_SG_D_2_52177 : Outport
  wires:
  Subtract_4d5aa/1 -> Product_cf416/2
  Constant_x_l_18580/1 -> Subtract_c1786/2
  Divide_f76fa/1 -> Add_e30b2/2
  Subtract_50a4c/1 -> Product_20c61/2
  Constant_-1_b3346/1 -> Product_802e4/1
  Constant_x_dd_b4462/1 -> Subtract_a8385/1
  Divide_4ce7a/1 -> Blockout_d_psi_1d_SG_D_2_52177/1
  State_psi_fd_SG_D_2_21e47/1 -> Add_8c972/2
  State_psi_1d_SG_D_2_6e6f3/1 -> Product_802e4/2
  Divide_4f7f4/1 -> Subtract_50a4c/2
  Constant_x_ddd_69af6/1 -> Subtract_a8385/2
  State_psi_1d_SG_D_2_7ee43/1 -> Product_4e370/2
  Product_802e4/1 -> Product_97c58/1
  Subtract_a8385/1 -> Product_97c58/2
  Constant_x_dd_70482/1 -> Subtract_c1786/1
  Constant_x_ddd_7a908/1 -> Subtract_4d5aa/1
  Constant_x_l_fd65c/1 -> Subtract_4d5aa/2
  Product_97c58/1 -> Divide_ed9f4/1
  Subtract_c1786/1 -> Divide_ed9f4/2
  State_psi_fd_SG_D_2_221ae/1 -> Product_cf416/1
  Constant_x_dd_0e8be/1 -> Subtract_0d414/1
  Constant_x_l_fe476/1 -> Subtract_f99a1/2
  Constant_x_l_3de7a/1 -> Subtract_0d414/2
  Constant_x_ddd_a8d87/1 -> Divide_f76fa/2
  Divide_ed9f4/1 -> Add_0985b/1
  State_psi_d_SG_D_2_2e599/1 -> Add_0985b/2
  Product_cf416/1 -> Divide_4f7f4/1
  Subtract_0d414/1 -> Divide_4f7f4/2
  Constant_x_dd_e3a6e/1 -> Subtract_f99a1/1
  Add_0985b/1 -> Subtract_50a4c/1
  Constant_-1_ac0c6/1 -> Product_4e370/1
  Subtract_f99a1/1 -> Product_20c61/1
  Product_4e370/1 -> Add_8c972/1
  Product_20c61/1 -> Divide_f76fa/1
  Add_8c972/1 -> Add_e30b2/1
  Add_e30b2/1 -> Divide_4ce7a/1
  Constant_T_ddd_fa46a/1 -> Divide_4ce7a/2
